simulink library "seriallib"  (Simulink 5.0)
undefined symbols (not defined in the file or in its folder): mbaseserialmask, mmodemcontrol, mquamask, mrs232
libraries: xpclib x193, vxlib x36, simulink x4
(part 2 of 3)

== system seriallib/RS232/Quatech/QSC-200/300 ==
  Modem Control : S-Function  InitFcn=mmodemcontrol(3)  FunctionName=modemcontrolqua  Parameters=slot, port, boardtype, rts, dtr, count  mask(QSC-200/300 Modem Control){port=1, rts=on, dtr=on, slot=-1}
      mask prompts: slot "PCI slot: (-1 for autosearch)"
      mask help:
      | QSC-200/300
      | Quatech
      | Modem Control
      mask init:
      | count = 0;
      | boardtype = 3;
      | [maskdisplay, count] = mmodemcontrol( 2, rts, dtr, boardtype, 0, 0 );
      | set_param( gcb, 'MaskDisplay', maskdisplay );
      mask Help: helpview(fullfile(docroot, 'mapfiles', 'xpc.map'), 'Quatech_MODEM_Control')
      mask StyleString: popup(1|2|3|4),checkbox,checkbox,edit
      mask Display: disp('QSC-200/300\nQuatech\nModem Control');port_label('input',1,'RTS');port_label('input',2,'DTR');
  Modem Status : S-Function  FunctionName=modemstatusqua  Parameters=slot, port, boardtype, cts, dsr, ring, dcd, count, sampletime  mask(Modem Status){port=1, cts=on, dsr=on, ring=on, dcd=on, sampletime=-1, slot=-1}
      mask prompts: ring "RI:"; slot "PCI slot: (-1 for autosearch)"
      mask help:
      | QSC-200/300
      | Quatech
      | Modem Status
      mask init:
      | count = 0;
      | boardtype = 3;
      | [maskdisplay, count] = mmodemstatus( 2, cts, dsr, ring, dcd, boardtype );
      | set_param( gcb, 'MaskDisplay', maskdisplay );
      mask Help: helpview(fullfile(docroot, 'mapfiles', 'xpc.map'), 'Quatech_MODEM_Status')
      mask StyleString: popup(1|2|3|4),checkbox,checkbox,checkbox,checkbox,edit,edit
      mask Display: disp('QSC-200/300\nQuatech\nModem Status');port_label('output',1,'CTS');port_label('output',2,'DSR');port_label('output',3,'RI');port_label('output',4,'DCD');
  QSC-200/300 Internal  blocks1 : Subsystem
  "QSC-200/300 " : Subsystem  InitFcn=mquamask(3)  TreatAsAtomicUnit=on  mask(RS422/485 Send Receive){group=Board Setup, port=1, irqnum=7, slot=-1, baud1=115200, parity1=None, ndata1=8, nstop1=1, fifomode1=64 deep, rlevel1=half full, onxmt1=None, xmtfifosize1=1024, xmtdatatype1=8 bit uint null terminated, rcvfifosize1=1024, rcvmaxread1=1024, rcvminread1=1, rcvusedelim1=on, rcvdelim1=13, rcvdatatype1=count+16 bit uint, rcvsampletime1=-1, baud2=115200, parity2=None, ndata2=8, nstop2=1, fifomode2=64 deep, rlevel2=half full, onxmt2=None, xmtfifosize2=1024, xmtdatatype2=8 bit uint null terminated, rcvfifosize2=1024, rcvmaxread2=1024, rcvminread2=1, rcvusedelim2=on, rcvdelim2=13, rcvdatatype2=count+16 bit uint, rcvsampletime2=-1, baud3=115200, parity3=None, ndata3=8, nstop3=1, fifomode3=64 deep, rlevel3=half full, onxmt3=None, xmtfifosize3=1024, xmtdatatype3=8 bit uint null terminated, rcvfifosize3=1024, rcvmaxread3=1024, rcvminread3=1, rcvusedelim3=on, rcvdelim3=13, rcvdatatype3=count+16 bit uint, rcvsampletime3=-1, buad4=115200, parity4=None, ndata4=8, nstop4=1, fifomode4=64 deep, rlevel4=half full, onxmt4=None, xmtfifosize4=1024, xmtdatatype4=8 bit uint null terminated, rcvfifosize4=1024, rcvmaxread4=1024, rcvminread4=1, rcvusedelim4=on, rcvdelim4=13, rcvdatatype4=count+16 bit uint, rcvsampletime4=-1}
      mask prompts: group "Parameter group:"; port "Port to modify:"; irqnum "IRQ number:"; baud1 "Baud rate:"; parity1 "Parity:"; ndata1 "Data bits:"; nstop1 "Stop bits:"; fifomode1 "Hardware fifo size:"; rlevel1 "Receive fifo interrupt level:"; onxmt1 "Assert on transmit:"; xmtfifosize1 "Transmit software fifo size:"; xmtdatatype1 "Transmit fifo data type:"; rcvfifosize1 "Receive software fifo size:"; rcvmaxread1 "Receive maximum read:"; rcvminread1 "Receive minimum read:"; rcvusedelim1 "Read to delimiter:"; rcvdelim1 "Delimiter:"; rcvdatatype1 "Receive data type:"; rcvsampletime1 "Receive SampleTime:"; baud2 "Baud rate:"; parity2 "Parity:"; ndata2 "Data bits:"; nstop2 "Stop bits:"; fifomode2 "Hardware fifo size:"; rlevel2 "Receive fifo interrupt level:"; onxmt2 "Assert on transmit:"; xmtfifosize2 "Transmit software fifo size:"; xmtdatatype2 "Transmit fifo data type:"; rcvfifosize2 "Receive software fifo size:"; rcvmaxread2 "Receive maximum read:"; rcvminread2 "Receive minimum read:"; rcvusedelim2 "Read to delimiter:"; rcvdelim2 "Delimiter:"; rcvdatatype2 "Receive data type:"; rcvsampletime2 "Receive SampleTime:"; baud3 "Baud rate:"; parity3 "Parity:"; ndata3 "Data bits:"; nstop3 "Stop bits:"; fifomode3 "Hardware fifo size:"; rlevel3 "Receive fifo interrupt level:"; onxmt3 "Assert on transmit:"; xmtfifosize3 "Transmit software fifo size:"; xmtdatatype3 "Transmit fifo data type:"; rcvfifosize3 "Receive software fifo size:"; rcvmaxread3 "Receive maximum read:"; rcvminread3 "Receive minimum read:"; rcvusedelim3 "Read to delimiter:"; rcvdelim3 "Delimiter:"; rcvdatatype3 "Receive data type:"; rcvsampletime3 "Receive SampleTime:"; buad4 "Baud rate:"; parity4 "Parity:"; ndata4 "Data bits:"; nstop4 "Stop bits:"; fifomode4 "Hardware fifo size:"; rlevel4 "Receive fifo interrupt level:"; onxmt4 "Assert on transmit:"; xmtfifosize4 "Transmit software fifo size:"; xmtdatatype4 "Transmit fifo data type:"; rcvfifosize4 "Receive software fifo size:"; rcvmaxread4 "Receive maximum read:"; rcvminread4 "Receive minimum read:"; rcvusedelim4 "Read to delimiter:"; rcvdelim4 "Delimiter:"; rcvdatatype4 "Receive data type:"; rcvsampletime4 "Receive SampleTime:"
      mask help:
      | QSC-200/300
      | Quatech
      | RS422/485 Send Receive Subsystem
      mask init:
      | brdslot = slot;
      | mqua2mask( 1, 4 );
      mask Help: helpview(fullfile(docroot, 'mapfiles', 'xpc.map'), 'Quatech_Subsystem')
      mask StyleString: popup(Board Setup|Basic Setup|Transmit Setup|Receive Setup),popup(1|2|3|4),edit,edit,popup(921600|460800|230400|115200|57600|38400|19200|9600|4800|2400|1200|600|300|110),popup(None|Even|Odd|Mark|Space),popup(5|6|7|8),popup(1|2),popup(64 deep|16 deep|1 deep),popup(1|quarter full|half full|almost full),popup(None|RTS|DTR),edit,popup(count+32 bit int|count+32 bit uint|count+16 bit int|count+16 bit uint|8 bit int null terminated|8 bit uint null terminated),edit,edit,edit,checkbox,edit,popup(count+32 bit int|count+32 bit uint|count+16 bit int|count+16 bit uint|8 bit int null terminated|8 bit uint null terminated),edit,popup(921600|460800|230400|115200|57600|38400|19200|9600|4800|2400|1200|600|300|110),popup(None|Even|Odd|Mark|Space),popup(5|6|7|8),popup(1|2),popup(64 deep|16 deep|1 deep),popup(1|quarter full|half full|almost full),popup(None|RTS|DTR),edit,popup(count+32 bit int|count+32 bit uint|count+16 bit int|count+16 bit uint|8 bit int null terminated|8 bit uint null terminated),edit,edit,edit,checkbox,edit,popup(count+32 bit int|count+32 bit uint|count+16 bit int|count+16 bit uint|8 bit int null terminated|8 bit uint null terminated),edit,popup(921600|460800|230400|115200|57600|38400|19200|9600|4800|2400|1200|600|300|110),popup(None|Even|Odd|Mark|Space),popup(5|6|7|8),popup(1|2),popup(64 deep|16 deep|1 deep),popup(1|quarter full|half full|almost full),popup(None|RTS|DTR),edit,popup(count+32 bit int|count+32 bit uint|count+16 bit int|count+16 bit uint|8 bit int null terminated|8 bit uint null terminated),edit,edit,edit,checkbox,edit,popup(count+32 bit int|count+32 bit uint|count+16 bit int|count+16 bit uint|8 bit int null terminated|8 bit uint null terminated),edit,popup(921600|460800|230400|115200|57600|38400|19200|9600|4800|2400|1200|600|300|110),popup(None|Even|Odd|Mark|Space),popup(5|6|7|8),popup(1|2),popup(64 deep|16 deep|1 deep),popup(1|quarter full|half full|almost full),popup(None|RTS|DTR),edit,popup(count+32 bit int|count+32 bit uint|count+16 bit int|count+16 bit uint|8 bit int null terminated|8 bit uint null terminated),edit,edit,edit,checkbox,edit,popup(count+32 bit int|count+32 bit uint|count+16 bit int|count+16 bit uint|8 bit int null terminated|8 bit uint null terminated),edit
      mask CallbackString:
      | mquamask( 2, 4 );
      | |mquamask( 2, 4 );||||||||||||||||||||||||||||||||||||||||||||||||||||||||||||||||||
      mask Display:
      | disp('QSC-200/300\n\nRS422/485\n\nSend Receive');
      | port_label( 'input', 1, 'XMT1' );
      | port_label( 'input', 2, 'XMT2' );
      | port_label( 'input', 3, 'XMT3' );
      | port_label( 'input', 4, 'XMT4' );
      | port_label( 'output', 1, 'RCV1' );
      | port_label( 'output', 2, 'RCV2' );
      | port_label( 'output', 3, 'RCV3' );
      | port_label( 'output', 4, 'RCV4' );

== system seriallib/RS232/Synchronous Mode/Send & Receive  ==
  In1 : Inport
  S-Function : S-Function  FunctionName=rs232_sendrec  Parameters=port,formatsend,formatrec,numb,ts
  Out1 : Outport
  wires:
  S-Function/1 -> Out1/1
  In1/1 -> S-Function/1

== system seriallib/RS232/Mainboard/Baseboard Serial/RS232 ISR ==
  Xmt 1 : Inport
  Xmt 2 : Inport  Port=2
  function : TriggerPort  TriggerType=function-call
  While Iterator Subsystem : Subsystem  TreatAsAtomicUnit=on
  Recv 1 : Outport
  Recv 2 : Outport  Port=2
  wires:
  While Iterator Subsystem/2(Recv 2) -> Recv 2/1
  While Iterator Subsystem/1(Recv 1) -> Recv 1/1
  Xmt 2/1 -> While Iterator Subsystem/2(Xmt 2)
  Xmt 1/1 -> While Iterator Subsystem/1(Xmt 1)

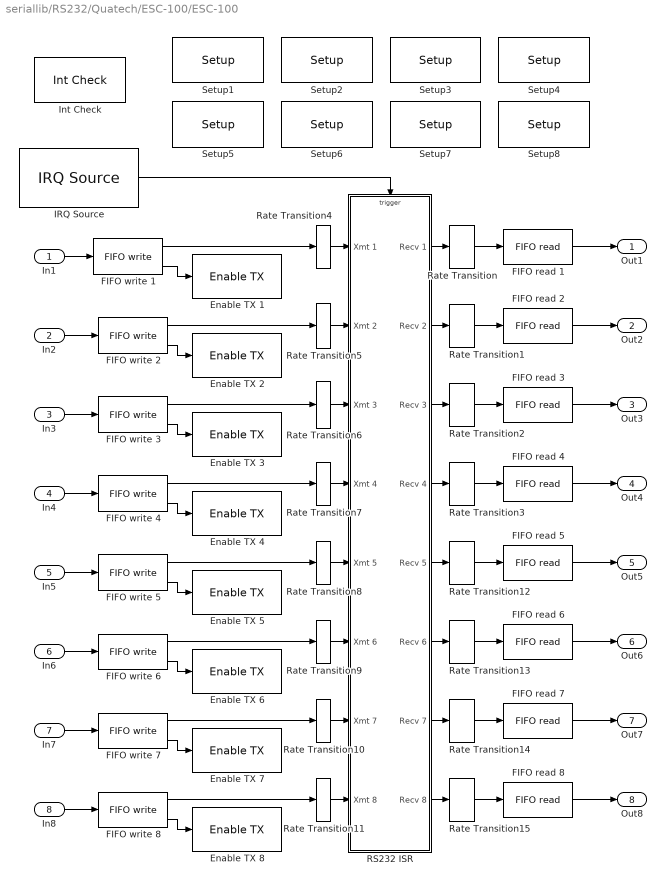
== system seriallib/RS232/Quatech/ESC-100/ESC-100 ==
  In1 : Inport
  In2 : Inport  Port=2
  In3 : Inport  Port=3
  In4 : Inport  Port=4
  In5 : Inport  Port=5
  In6 : Inport  Port=6
  In7 : Inport  Port=7
  In8 : Inport  Port=8
  Enable TX 1 : xpclib/RS232/Quatech/ESC-100/ESC-100 Internal blocks/Enable TX   port=1  slot=brdslot
  Enable TX 2 : xpclib/RS232/Quatech/ESC-100/ESC-100 Internal blocks/Enable TX   port=2  slot=brdslot
  Enable TX 3 : xpclib/RS232/Quatech/ESC-100/ESC-100 Internal blocks/Enable TX   port=3  slot=brdslot
  Enable TX 4 : xpclib/RS232/Quatech/ESC-100/ESC-100 Internal blocks/Enable TX   port=4  slot=brdslot
  Enable TX 5 : xpclib/RS232/Quatech/ESC-100/ESC-100 Internal blocks/Enable TX   port=5  slot=brdslot
  Enable TX 6 : xpclib/RS232/Quatech/ESC-100/ESC-100 Internal blocks/Enable TX   port=6  slot=brdslot
  Enable TX 7 : xpclib/RS232/Quatech/ESC-100/ESC-100 Internal blocks/Enable TX   port=7  slot=brdslot
  Enable TX 8 : xpclib/RS232/Quatech/ESC-100/ESC-100 Internal blocks/Enable TX   port=8  slot=brdslot
  FIFO read {1..8} (8 alike) : xpclib/RS232/FIFO read   maxsize=1024  minsize=1  usedelimiter=on  delimiter=13  outputtype=count+16 bit uint  enable=off  enableout=off  sampletime=-1
  FIFO write {1..8} (8 alike) : xpclib/RS232/FIFO write   size=1024  inputtype=8 bit uint null terminated  present=on  sampletime=-1
  IRQ Source : xpclib/Asynchronous Event/IRQ Source  irqNo=7  preempt=off  b_type=None/Other  slot=brdslot
  Int Check : xpclib/RS232/Quatech/ESC-100/ESC-100 Internal blocks/Int Check  slot=brdslot  irqnum=7
  RS232 ISR : Subsystem  TreatAsAtomicUnit=on  mask(RS232 ISR){slot=brdslot}
      mask help:
      | ESC-100
      | Quatech
      | Interrupt Service Routine
      mask init:
      | subslot = slot;
      mask Display:
      | disp('ESC-100\nISR');
      | port_label('input', 1, 'XMT1');
      | port_label('input', 2, 'XMT2');
      | port_label('input', 3, 'XMT3');
      | port_label('input', 4, 'XMT4');
      | port_label('input', 5, 'XMT5');
      | port_label('input', 6, 'XMT6');
      | port_label('input', 7, 'XMT7');
      | port_label('input', 8, 'XMT8');
      | port_label('output', 1, 'RCV1');
      | port_label('output', 2, 'RCV2');
      | port_label('output', 3, 'RCV3');
      | port_label('output', 4, 'RCV4');
      | port_label('output', 5, 'RCV5');
      | port_label('output', 6, 'RCV6');
      | port_label('output', 7, 'RCV7');
      | port_label('output', 8, 'RCV8');
  Rate Transition{,1..15} (16 alike) : vxlib/Asynchronous Support/Rate Transition  sample_time=-1
  Setup1 : xpclib/RS232/Quatech/ESC-100/ESC-100 Internal blocks/Setup  port=1  baud=19200  width=8  nstop=1  parity=None  fmode=64 deep  rlevel=half full  ctsmode=on  slot=brdslot
  Setup2 : xpclib/RS232/Quatech/ESC-100/ESC-100 Internal blocks/Setup  port=2  baud=19200  width=8  nstop=1  parity=None  fmode=64 deep  rlevel=half full  ctsmode=on  slot=brdslot
  Setup3 : xpclib/RS232/Quatech/ESC-100/ESC-100 Internal blocks/Setup  port=3  baud=19200  width=8  nstop=1  parity=None  fmode=64 deep  rlevel=half full  ctsmode=on  slot=brdslot
  Setup4 : xpclib/RS232/Quatech/ESC-100/ESC-100 Internal blocks/Setup  port=4  baud=19200  width=8  nstop=1  parity=None  fmode=64 deep  rlevel=half full  ctsmode=on  slot=brdslot
  Setup5 : xpclib/RS232/Quatech/ESC-100/ESC-100 Internal blocks/Setup  port=5  baud=19200  width=8  nstop=1  parity=None  fmode=64 deep  rlevel=half full  ctsmode=on  slot=brdslot
  Setup6 : xpclib/RS232/Quatech/ESC-100/ESC-100 Internal blocks/Setup  port=6  baud=19200  width=8  nstop=1  parity=None  fmode=64 deep  rlevel=half full  ctsmode=on  slot=brdslot
  Setup7 : xpclib/RS232/Quatech/ESC-100/ESC-100 Internal blocks/Setup  port=7  baud=19200  width=8  nstop=1  parity=None  fmode=64 deep  rlevel=half full  ctsmode=on  slot=brdslot
  Setup8 : xpclib/RS232/Quatech/ESC-100/ESC-100 Internal blocks/Setup  port=8  baud=19200  width=8  nstop=1  parity=None  fmode=64 deep  rlevel=half full  ctsmode=on  slot=brdslot
  Out1 : Outport
  Out2 : Outport  Port=2
  Out3 : Outport  Port=3
  Out4 : Outport  Port=4
  Out5 : Outport  Port=5
  Out6 : Outport  Port=6
  Out7 : Outport  Port=7
  Out8 : Outport  Port=8
  wires:
  In8/1 -> FIFO write 8/1
  In7/1 -> FIFO write 7/1
  In6/1 -> FIFO write 6/1
  In5/1 -> FIFO write 5/1
  In4/1 -> FIFO write 4/1
  In3/1 -> FIFO write 3/1
  In2/1 -> FIFO write 2/1
  FIFO write 8/2 -> Enable TX 8/1
  FIFO write 7/2 -> Enable TX 7/1
  FIFO write 6/2 -> Enable TX 6/1
  FIFO write 5/2 -> Enable TX 5/1
  FIFO write 4/2 -> Enable TX 4/1
  FIFO write 3/2 -> Enable TX 3/1
  FIFO write 2/2 -> Enable TX 2/1
  FIFO write 8/1 -> Rate Transition11/1
  FIFO write 7/1 -> Rate Transition10/1
  FIFO write 6/1 -> Rate Transition9/1
  FIFO write 5/1 -> Rate Transition8/1
  FIFO write 4/1 -> Rate Transition7/1
  FIFO write 3/1 -> Rate Transition6/1
  FIFO write 2/1 -> Rate Transition5/1
  FIFO write 1/2 -> Enable TX 1/1
  FIFO write 1/1 -> Rate Transition4/1
  In1/1 -> FIFO write 1/1
  IRQ Source/1 -> RS232 ISR/Trigger
  Rate Transition4/1 -> RS232 ISR/1(Xmt 1)
  Rate Transition6/1 -> RS232 ISR/3(Xmt 3)
  Rate Transition7/1 -> RS232 ISR/4(Xmt 4)
  RS232 ISR/1(Recv 1) -> Rate Transition/1
  RS232 ISR/2(Recv 2) -> Rate Transition1/1
  RS232 ISR/3(Recv 3) -> Rate Transition2/1
  Rate Transition/1 -> FIFO read 1/1
  FIFO read 1/1 -> Out1/1
  Rate Transition1/1 -> FIFO read 2/1
  FIFO read 2/1 -> Out2/1
  FIFO read 3/1 -> Out3/1
  FIFO read 4/1 -> Out4/1
  Rate Transition2/1 -> FIFO read 3/1
  Rate Transition3/1 -> FIFO read 4/1
  Rate Transition5/1 -> RS232 ISR/2(Xmt 2)
  RS232 ISR/4(Recv 4) -> Rate Transition3/1
  Rate Transition11/1 -> RS232 ISR/8(Xmt 8)
  Rate Transition10/1 -> RS232 ISR/7(Xmt 7)
  Rate Transition9/1 -> RS232 ISR/6(Xmt 6)
  Rate Transition8/1 -> RS232 ISR/5(Xmt 5)
  FIFO read 5/1 -> Out5/1
  Rate Transition12/1 -> FIFO read 5/1
  FIFO read 6/1 -> Out6/1
  Rate Transition13/1 -> FIFO read 6/1
  FIFO read 7/1 -> Out7/1
  Rate Transition14/1 -> FIFO read 7/1
  FIFO read 8/1 -> Out8/1
  Rate Transition15/1 -> FIFO read 8/1
  RS232 ISR/5(Recv 5) -> Rate Transition12/1
  RS232 ISR/6(Recv 6) -> Rate Transition13/1
  RS232 ISR/7(Recv 7) -> Rate Transition14/1
  RS232 ISR/8(Recv 8) -> Rate Transition15/1

== system seriallib/RS232/Quatech/ESC-100/ESC-100 Internal blocks ==
  "Enable TX " : S-Function  FunctionName=sertxenable  Parameters=slot, port, 2  mask(Enable TX Int){port=1, slot=-1}
      mask prompts: slot "PCI slot: (-1 for autosearch)"
      mask help:
      | ESC-100
      | Quatech
      | Enable TX Interrupt
      mask Help: helpview(fullfile(docroot, 'mapfiles', 'xpc.map'), 'Quatech_Enable_Int')
      mask StyleString: popup(1|2|3|4|5|6|7|8),edit
      mask Display:
      | disp('ESC-100\nQuatech\nEnable TX int');
      | port_label('input', 1, 'E');
  Filter Int Reason : S-Function  FunctionName=filterqua  Parameters=port, 2, value  mask(Interrupt Source Filter){port=1, value=Transmitter empty}
      mask prompts: value "Filter value:"
      mask help:
      | ESC-100
      | Quatech
      | Interrupt Source Filter
      mask Help: helpview(fullfile(docroot, 'mapfiles', 'xpc.map'), 'Quatech_Filter_Ints')
      mask StyleString: popup(1|2|3|4|5|6|7|8),popup(Receive data|Transmitter empty|Modem status change)
      mask Display:
      | disp('ESC-100\nQuatech\nFilter Int Reason');
      | port_label('input', 1, 'S' );
      | port_label('output', 1, 'E' );
  Int Check : S-Function  FunctionName=intcheckqua  Parameters=slot, irqnum+4, boardtype,  mask(interrupt check){slot=-1, irqnum=5}
      mask prompts: slot "PCI slot: (-1 for autosearch)"; irqnum "IRQ Line Number"
      mask help:
      | ESC-100
      | Quatech
      | Interrupt Check
      mask init:
      | boardtype = 2;
      mask Help: helpview(fullfile(docroot, 'mapfiles', 'xpc.map'), 'Quatech_Interrupt_Check')
      mask StyleString: edit,popup(5|6|7|8|9|10|11|12|13|14|15)
      mask Display: disp('ESC-100\nQuatech\nInterrupt Check');
  Read HW FIFO : S-Function  FunctionName=serreadqua  Parameters=slot, port, 2, flush  mask(Read Data Port){port=1, flush=on, slot=-1}
      mask prompts: flush "Flush HW FIFO on startup"; slot "PCI slot: (-1 for autosearch)"
      mask help:
      | ESC-100
      | Quatech
      | Read Data Port
      mask Help: helpview(fullfile(docroot, 'mapfiles', 'xpc.map'), 'Quatech_Read_HW')
      mask StyleString: popup(1|2|3|4|5|6|7|8),checkbox,edit
      mask Display:
      | disp('ESC-100\nQuatech\nRead HW FIFO');
      | port_label('input', 1, 'E');
      | port_label('output', 1, 'D');
  Read Int Status : S-Function  FunctionName=Iqueryqua  Parameters=slot, 2  mask(Interrupt Query){slot=-1}
      mask prompts: slot "PCI slot: (-1 for autosearch)"
      mask help:
      | ESC-100
      | Quatech
      | Interrupt Query
      mask Help: helpview(fullfile(docroot, 'mapfiles', 'xpc.map'), 'Quatech_Interrupt_Query')
      mask Display:
      | disp('ESC-100\nQuatech\nRead Int Status');
      | port_label('output', 1, 'S' );
  Setup : S-Function  FunctionName=setupqua  Parameters=slot, boardtype, port, baud, width, nstop, parity, fmode, ctsmode, rlevel  mask(setup){port=1, baud=115200, width=8, nstop=1, parity=None, fmode=64 deep, rlevel=half full, ctsmode=off, slot=-1}
      mask prompts: baud "Baud rate:"; width "Number of data bits:"; nstop "Number of stop bits:"; fmode "Fifo mode:"; rlevel "Receive trigger level:"; ctsmode "Enable auto RTS/CTS"; slot "PCI slot: (-1 for autosearch)"
      mask help:
      | ESC-100
      | Quatech
      | Setup
      mask init:
      | boardtype = 2;
      mask Help: helpview(fullfile(docroot, 'mapfiles', 'xpc.map'), 'Quatech_Setup')
      mask StyleString: popup(1|2|3|4|5|6|7|8),popup(921600|460800|230400|115200|57600|38400|19200|9600|4800|2400|1200|600|300|110),popup(5|6|7|8),popup(1|2),popup(None|Even|Odd|Mark|Space),popup(64 deep|16 deep|1 deep),popup(1|quarter full|half full|almost full),checkbox,edit
      mask Display: disp('ESC-100\nQuatech\nSetup')
  Write HW FIFO : S-Function  FunctionName=serwritequa  Parameters=slot, port, 2, 0  mask(Write Data Port){port=1, slot=-1}
      mask prompts: slot "PCI slot: (-1 for autosearch)"
      mask help:
      | ESC-100
      | Quatech
      | Write Data Port
      mask Help: helpview(fullfile(docroot, 'mapfiles', 'xpc.map'), 'Quatech_Write_HW')
      mask StyleString: popup(1|2|3|4|5|6|7|8),edit
      mask Display:
      | disp('ESC-100\nQuatech\nWrite HW FIFO');
      | port_label('input', 1, 'D');
      | port_label('input', 2, 'E');

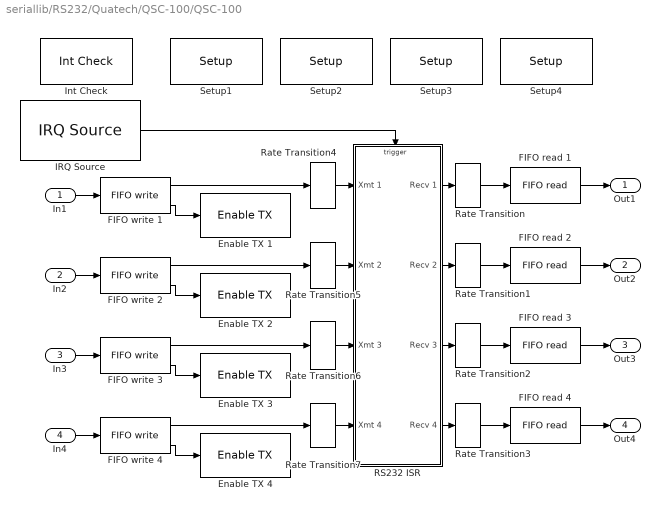
== system seriallib/RS232/Quatech/QSC-100/QSC-100 ==
  In1 : Inport
  In2 : Inport  Port=2
  In3 : Inport  Port=3
  In4 : Inport  Port=4
  Enable TX 1 : xpclib/RS232/Quatech/QSC-100/QSC-100 Internal  blocks/Enable TX   port=1  slot=brdslot
  Enable TX 2 : xpclib/RS232/Quatech/QSC-100/QSC-100 Internal  blocks/Enable TX   port=2  slot=brdslot
  Enable TX 3 : xpclib/RS232/Quatech/QSC-100/QSC-100 Internal  blocks/Enable TX   port=3  slot=brdslot
  Enable TX 4 : xpclib/RS232/Quatech/QSC-100/QSC-100 Internal  blocks/Enable TX   port=4  slot=brdslot
  FIFO read {1..4} (4 alike) : xpclib/RS232/FIFO read   maxsize=1024  minsize=1  usedelimiter=on  delimiter=13  outputtype=count+16 bit uint  enable=off  enableout=off  sampletime=-1
  FIFO write {1..4} (4 alike) : xpclib/RS232/FIFO write   size=1024  inputtype=8 bit uint null terminated  present=on  sampletime=-1
  IRQ Source : xpclib/Asynchronous Event/IRQ Source  irqNo=7  preempt=off  b_type=None/Other  slot=brdslot
  Int Check : xpclib/RS232/Quatech/QSC-100/QSC-100 Internal  blocks/Int Check  slot=brdslot  irqnum=7
  RS232 ISR : Subsystem  TreatAsAtomicUnit=on  mask(RS232 ISR){slot=brdslot}
      mask help:
      | QSC-100
      | Quatech
      | Interrupt Service Routine
      mask init:
      | subslot = slot;
      mask Display:
      | disp('QSC-100\nISR');
      | port_label('input', 1, 'XMT1');
      | port_label('input', 2, 'XMT2');
      | port_label('input', 3, 'XMT3');
      | port_label('input', 4, 'XMT4');
      | port_label('output', 1, 'RCV1');
      | port_label('output', 2, 'RCV2');
      | port_label('output', 3, 'RCV3');
      | port_label('output', 4, 'RCV4');
  Rate Transition{,1..7} (8 alike) : vxlib/Asynchronous Support/Rate Transition  sample_time=-1
  Setup1 : xpclib/RS232/Quatech/QSC-100/QSC-100 Internal  blocks/Setup  port=1  baud=115200  width=8  nstop=1  parity=None  fmode=64 deep  rlevel=half full  ctsmode=on  slot=brdslot
  Setup2 : xpclib/RS232/Quatech/QSC-100/QSC-100 Internal  blocks/Setup  port=2  baud=115200  width=8  nstop=1  parity=None  fmode=64 deep  rlevel=half full  ctsmode=on  slot=brdslot
  Setup3 : xpclib/RS232/Quatech/QSC-100/QSC-100 Internal  blocks/Setup  port=3  baud=115200  width=8  nstop=1  parity=None  fmode=64 deep  rlevel=half full  ctsmode=on  slot=brdslot
  Setup4 : xpclib/RS232/Quatech/QSC-100/QSC-100 Internal  blocks/Setup  port=4  baud=115200  width=8  nstop=1  parity=None  fmode=64 deep  rlevel=half full  ctsmode=on  slot=brdslot
  Out1 : Outport
  Out2 : Outport  Port=2
  Out3 : Outport  Port=3
  Out4 : Outport  Port=4
  wires:
  RS232 ISR/4(Recv 4) -> Rate Transition3/1
  Rate Transition5/1 -> RS232 ISR/2(Xmt 2)
  FIFO write 4/2 -> Enable TX 4/1
  FIFO write 3/2 -> Enable TX 3/1
  FIFO write 2/2 -> Enable TX 2/1
  Rate Transition3/1 -> FIFO read 4/1
  Rate Transition2/1 -> FIFO read 3/1
  FIFO read 4/1 -> Out4/1
  FIFO read 3/1 -> Out3/1
  FIFO read 2/1 -> Out2/1
  Rate Transition1/1 -> FIFO read 2/1
  FIFO read 1/1 -> Out1/1
  Rate Transition/1 -> FIFO read 1/1
  In2/1 -> FIFO write 2/1
  In3/1 -> FIFO write 3/1
  In4/1 -> FIFO write 4/1
  FIFO write 4/1 -> Rate Transition7/1
  FIFO write 3/1 -> Rate Transition6/1
  FIFO write 2/1 -> Rate Transition5/1
  In1/1 -> FIFO write 1/1
  FIFO write 1/1 -> Rate Transition4/1
  RS232 ISR/3(Recv 3) -> Rate Transition2/1
  RS232 ISR/2(Recv 2) -> Rate Transition1/1
  RS232 ISR/1(Recv 1) -> Rate Transition/1
  Rate Transition7/1 -> RS232 ISR/4(Xmt 4)
  Rate Transition6/1 -> RS232 ISR/3(Xmt 3)
  Rate Transition4/1 -> RS232 ISR/1(Xmt 1)
  IRQ Source/1 -> RS232 ISR/Trigger
  FIFO write 1/2 -> Enable TX 1/1

== system seriallib/RS232/Quatech/QSC-100/QSC-100 Internal  blocks ==
  "Enable TX " : S-Function  FunctionName=sertxenable  Parameters=slot, port, 1  mask(Enable TX Int){port=1, slot=-1}
      mask prompts: slot "PCI slot: (-1 for autosearch)"
      mask help:
      | QSC-100
      | Quatech
      | Enable TX Interrupt
      mask Help: helpview(fullfile(docroot, 'mapfiles', 'xpc.map'), 'Quatech_Enable_Int')
      mask StyleString: popup(1|2|3|4),edit
      mask Display:
      | disp('QSC-100\nQuatech\nEnable TX int');
      | port_label('input', 1, 'E');
  Filter Int Reason : S-Function  FunctionName=filterqua  Parameters=port, 1, value  mask(Interrupt Source Filter){port=1, value=Receive data}
      mask prompts: value "Filter value:"
      mask help:
      | QSC-100
      | Quatech
      | Interrupt Source Filter
      mask Help: helpview(fullfile(docroot, 'mapfiles', 'xpc.map'), 'Quatech_Filter_Ints')
      mask StyleString: popup(1|2|3|4),popup(Receive data|Transmitter empty|Modem status change)
      mask Display:
      | disp('QSC-100\nQuatech\nFilter Int Reason');
      | port_label('input', 1, 'S' );
      | port_label('output', 1, 'E' );
  Int Check : S-Function  FunctionName=intcheckqua  Parameters=slot, irqnum+4, boardtype,  mask(interrupt check){slot=-1, irqnum=5}
      mask prompts: slot "PCI slot: (-1 for autosearch)"; irqnum "IRQ Line Number"
      mask help:
      | QSC-100
      | Quatech
      | Interrupt Check
      mask init:
      | boardtype = 1;
      mask Help: helpview(fullfile(docroot, 'mapfiles', 'xpc.map'), 'Quatech_Interrupt_Check')
      mask StyleString: edit,popup(5|6|7|8|9|10|11|12|13|14|15)
      mask Display: disp('QSC-100\nQuatech\nInterrupt Check');
  Read HW FIFO : S-Function  FunctionName=serreadqua  Parameters=slot, port, 1, flush  mask(Read Data Port){port=1, flush=on, slot=-1}
      mask prompts: flush "Flush HW FIFO on startup"; slot "PCI slot: (-1 for autosearch)"
      mask help:
      | QSC-100
      | Quatech
      | Read Data Port
      mask Help: helpview(fullfile(docroot, 'mapfiles', 'xpc.map'), 'Quatech_Read_HW')
      mask StyleString: popup(1|2|3|4),checkbox,edit
      mask Display:
      | disp('QSC-100\nQuatech\nRead HW FIFO');
      | port_label('input', 1, 'E');
      | port_label('output', 1, 'D');
  Read Int Status : S-Function  FunctionName=Iqueryqua  Parameters=slot, 1  mask(Interrupt Query){slot=-1}
      mask prompts: slot "PCI slot: (-1 for autosearch)"
      mask help:
      | QSC-100
      | Quatech
      | Interrupt Query
      mask Help: helpview(fullfile(docroot, 'mapfiles', 'xpc.map'), 'Quatech_Interrupt_Query')
      mask Display:
      | disp('QSC-100\nQuatech\nRead Int Status');
      | port_label('output', 1, 'S' );
  Setup : S-Function  FunctionName=setupqua  Parameters=slot, boardtype, port, baud, width, nstop, parity, fmode, ctsmode, rlevel  mask(setup){port=1, baud=115200, width=8, nstop=1, parity=None, fmode=64 deep, rlevel=half full, ctsmode=off, slot=-1}
      mask prompts: baud "Baud rate:"; width "Number of data bits:"; nstop "Number of stop bits:"; fmode "Fifo mode:"; rlevel "Receive trigger level:"; ctsmode "Enable auto RTS/CTS"; slot "PCI slot: (-1 for autosearch)"
      mask help:
      | QSC-100
      | Quatech
      | Setup
      mask init:
      | boardtype = 1;
      mask Help: helpview(fullfile(docroot, 'mapfiles', 'xpc.map'), 'Quatech_Setup')
      mask StyleString: popup(1|2|3|4),popup(921600|460800|230400|115200|57600|38400|19200|9600|4800|2400|1200|600|300|110),popup(5|6|7|8),popup(1|2),popup(None|Even|Odd|Mark|Space),popup(64 deep|16 deep|1 deep),popup(1|quarter full|half full|almost full),checkbox,edit
      mask Display: disp('QSC-100\nQuatech\nSetup');
  Write HW FIFO : S-Function  FunctionName=serwritequa  Parameters=slot, port, 1, 0  mask(Write Data Port){port=1, slot=-1}
      mask prompts: slot "PCI slot: (-1 for autosearch)"
      mask help:
      | QSC-100
      | Quatech
      | Write Data Port
      mask Help: helpview(fullfile(docroot, 'mapfiles', 'xpc.map'), 'Quatech_Write_HW')
      mask StyleString: popup(1|2|3|4),edit
      mask Display:
      | disp('QSC-100\nQuatech\nWrite HW FIFO');
      | port_label('input', 1, 'D');
      | port_label('input', 2, 'E');

== system seriallib/RS232/Quatech/QSC-200/300/QSC-200/300 Internal  blocks1 ==
  "Enable TX " : S-Function  FunctionName=sertxenable  Parameters=slot, port, 3  mask(Enable TX Int){port=1, slot=-1}
      mask prompts: slot "PCI slot: (-1 for autosearch)"
      mask help:
      | QSC-200/300
      | Quatech
      | Enable TX Interrupt
      mask Help: helpview(fullfile(docroot, 'mapfiles', 'xpc.map'), 'Quatech_Enable_Int')
      mask StyleString: popup(1|2|3|4),edit
      mask Display:
      | disp('QSC-200/300\nQuatech\nEnable TX int');
      | port_label('input', 1, 'E');
  Filter Int Reason : S-Function  FunctionName=filterqua  Parameters=port, 3, value  mask(Interrupt Source Filter){port=1, value=Receive data}
      mask prompts: value "Filter value:"
      mask help:
      | QSC-200/300
      | Quatech
      | Interrupt Source Filter
      mask Help: helpview(fullfile(docroot, 'mapfiles', 'xpc.map'), 'Quatech_Filter_Ints')
      mask StyleString: popup(1|2|3|4),popup(Receive data|Transmitter empty|Modem status change)
      mask Display:
      | disp('QSC-200/300\nQuatech\nFilter Int Reason');
      | port_label('input', 1, 'S' );
      | port_label('output', 1, 'E' );
  Int Check : S-Function  FunctionName=intcheckqua  Parameters=slot, irqnum+4, boardtype,  mask(interrupt check){slot=-1, irqnum=5}
      mask prompts: slot "PCI slot: (-1 for autosearch)"; irqnum "IRQ Line Number"
      mask help:
      | QSC-200/300
      | Quatech
      | Interrupt Check
      mask init:
      | boardtype = 3;
      mask Help: helpview(fullfile(docroot, 'mapfiles', 'xpc.map'), 'Quatech_Interrupt_Check')
      mask StyleString: edit,popup(5|6|7|8|9|10|11|12|13|14|15)
      mask Display: disp('QSC-200/300\nQuatech\nInterrupt Check');
  Read HW FIFO : S-Function  FunctionName=serreadqua  Parameters=slot, port, 3, flush  mask(Read Data Port){port=1, flush=on, slot=-1}
      mask prompts: flush "Flush HW FIFO on startup"; slot "PCI slot: (-1 for autosearch)"
      mask help:
      | QSC-200/300
      | Quatech
      | Read Data Port
      mask Help: helpview(fullfile(docroot, 'mapfiles', 'xpc.map'), 'Quatech_Read_HW')
      mask StyleString: popup(1|2|3|4),checkbox,edit
      mask Display:
      | disp('QSC-200/300\nQuatech\nRead HW FIFO');
      | port_label('input', 1, 'E');
      | port_label('output', 1, 'D');
  Read Int Status : S-Function  FunctionName=Iqueryqua  Parameters=slot, 3  mask(Interrupt Query){slot=-1}
      mask prompts: slot "PCI slot: (-1 for autosearch)"
      mask help:
      | QSC-200/300
      | Quatech
      | Interrupt Query
      mask Help: helpview(fullfile(docroot, 'mapfiles', 'xpc.map'), 'Quatech_Interrupt_Query')
      mask Display:
      | disp('QSC-200/300\nQuatech\nRead Int Status');
      | port_label('output', 1, 'S' );
  Setup : S-Function  FunctionName=setupqua  Parameters=slot, boardtype, port, baud, width, nstop, parity, fmode, ctsmode, rlevel  mask(setup){port=1, baud=115200, width=8, nstop=1, parity=None, fmode=64 deep, rlevel=half full, ctsmode=off, slot=-1}
      mask prompts: baud "Baud rate:"; width "Number of data bits:"; nstop "Number of stop bits:"; fmode "Fifo mode:"; rlevel "Receive trigger level:"; ctsmode "Enable auto RTS/CTS"; slot "PCI slot: (-1 for autosearch)"
      mask help:
      | QSC-200/300
      | Quatech
      | Setup
      mask init:
      | boardtype = 3;
      mask Help: helpview(fullfile(docroot, 'mapfiles', 'xpc.map'), 'Quatech_Setup')
      mask StyleString: popup(1|2|3|4),popup(921600|460800|230400|115200|57600|38400|19200|9600|4800|2400|1200|600|300|110),popup(5|6|7|8),popup(1|2),popup(None|Even|Odd|Mark|Space),popup(64 deep|16 deep|1 deep),popup(1|quarter full|half full|almost full),checkbox,edit
      mask Display: disp('QSC-200/300\nQuatech\nSetup');
  Write HW FIFO : S-Function  FunctionName=serwritequa  Parameters=slot, port, 3, onxmt  mask(Write Data Port){port=1, onxmt=None, slot=-1}
      mask prompts: onxmt "Assert on Transmit:"; slot "PCI slot: (-1 for autosearch)"
      mask help:
      | QSC-200/300
      | Quatech
      | Write Data Port
      mask Help: helpview(fullfile(docroot, 'mapfiles', 'xpc.map'), 'Quatech_Write_HW')
      mask StyleString: popup(1|2|3|4),popup(None|RTS|DTR),edit
      mask Display:
      | disp('QSC-200/300\nQuatech\nWrite HW FIFO');
      | port_label('input', 1, 'D');
      | port_label('input', 2, 'E');

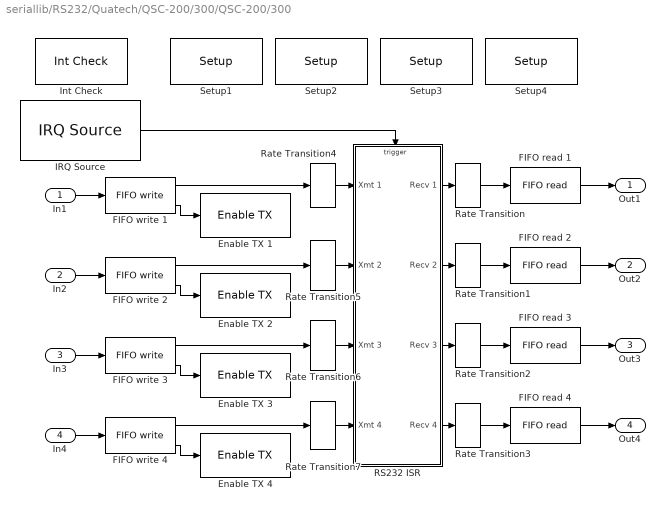
== system seriallib/RS232/Quatech/QSC-200/300/QSC-200/300  ==
  In1 : Inport
  In2 : Inport  Port=2
  In3 : Inport  Port=3
  In4 : Inport  Port=4
  Enable TX 1 : xpclib/RS232/Quatech/QSC-200//300/QSC-200//300 Internal  blocks1/Enable TX   port=1  slot=brdslot
  Enable TX 2 : xpclib/RS232/Quatech/QSC-200//300/QSC-200//300 Internal  blocks1/Enable TX   port=2  slot=brdslot
  Enable TX 3 : xpclib/RS232/Quatech/QSC-200//300/QSC-200//300 Internal  blocks1/Enable TX   port=3  slot=brdslot
  Enable TX 4 : xpclib/RS232/Quatech/QSC-200//300/QSC-200//300 Internal  blocks1/Enable TX   port=4  slot=brdslot
  FIFO read {1..4} (4 alike) : xpclib/RS232/FIFO read   maxsize=1024  minsize=1  usedelimiter=on  delimiter=13  outputtype=count+16 bit uint  enable=off  enableout=off  sampletime=-1
  FIFO write {1..4} (4 alike) : xpclib/RS232/FIFO write   size=1024  inputtype=8 bit uint null terminated  present=on  sampletime=-1
  IRQ Source : xpclib/Asynchronous Event/IRQ Source  irqNo=7  preempt=off  b_type=None/Other  slot=brdslot
  Int Check : xpclib/RS232/Quatech/QSC-200//300/QSC-200//300 Internal  blocks1/Int Check  slot=brdslot  irqnum=7
  RS232 ISR : Subsystem  TreatAsAtomicUnit=on  mask(RS232 ISR){slot=brdslot}
      mask help:
      | QSC-100
      | Quatech
      | Interrupt Service Routine
      mask init:
      | subslot = slot;
      mask Display:
      | disp('QSC-100\nISR');
      | port_label('input', 1, 'XMT1');
      | port_label('input', 2, 'XMT2');
      | port_label('input', 3, 'XMT3');
      | port_label('input', 4, 'XMT4');
      | port_label('output', 1, 'RCV1');
      | port_label('output', 2, 'RCV2');
      | port_label('output', 3, 'RCV3');
      | port_label('output', 4, 'RCV4');
  Rate Transition{,1..7} (8 alike) : vxlib/Asynchronous Support/Rate Transition  sample_time=-1
  Setup1 : xpclib/RS232/Quatech/QSC-200//300/QSC-200//300 Internal  blocks1/Setup  port=1  baud=115200  width=8  nstop=1  parity=None  fmode=64 deep  rlevel=half full  ctsmode=on  slot=brdslot
  Setup2 : xpclib/RS232/Quatech/QSC-200//300/QSC-200//300 Internal  blocks1/Setup  port=2  baud=115200  width=8  nstop=1  parity=None  fmode=64 deep  rlevel=half full  ctsmode=on  slot=brdslot
  Setup3 : xpclib/RS232/Quatech/QSC-200//300/QSC-200//300 Internal  blocks1/Setup  port=3  baud=115200  width=8  nstop=1  parity=None  fmode=64 deep  rlevel=half full  ctsmode=on  slot=brdslot
  Setup4 : xpclib/RS232/Quatech/QSC-200//300/QSC-200//300 Internal  blocks1/Setup  port=4  baud=115200  width=8  nstop=1  parity=None  fmode=64 deep  rlevel=half full  ctsmode=on  slot=brdslot
  Out1 : Outport
  Out2 : Outport  Port=2
  Out3 : Outport  Port=3
  Out4 : Outport  Port=4
  wires:
  FIFO write 1/2 -> Enable TX 1/1
  IRQ Source/1 -> RS232 ISR/Trigger
  Rate Transition4/1 -> RS232 ISR/1(Xmt 1)
  Rate Transition6/1 -> RS232 ISR/3(Xmt 3)
  Rate Transition7/1 -> RS232 ISR/4(Xmt 4)
  RS232 ISR/1(Recv 1) -> Rate Transition/1
  RS232 ISR/2(Recv 2) -> Rate Transition1/1
  RS232 ISR/3(Recv 3) -> Rate Transition2/1
  FIFO write 1/1 -> Rate Transition4/1
  In1/1 -> FIFO write 1/1
  FIFO write 2/1 -> Rate Transition5/1
  FIFO write 3/1 -> Rate Transition6/1
  FIFO write 4/1 -> Rate Transition7/1
  In4/1 -> FIFO write 4/1
  In3/1 -> FIFO write 3/1
  In2/1 -> FIFO write 2/1
  Rate Transition/1 -> FIFO read 1/1
  FIFO read 1/1 -> Out1/1
  Rate Transition1/1 -> FIFO read 2/1
  FIFO read 2/1 -> Out2/1
  FIFO read 3/1 -> Out3/1
  FIFO read 4/1 -> Out4/1
  Rate Transition2/1 -> FIFO read 3/1
  Rate Transition3/1 -> FIFO read 4/1
  FIFO write 2/2 -> Enable TX 2/1
  FIFO write 3/2 -> Enable TX 3/1
  FIFO write 4/2 -> Enable TX 4/1
  Rate Transition5/1 -> RS232 ISR/2(Xmt 2)
  RS232 ISR/4(Recv 4) -> Rate Transition3/1

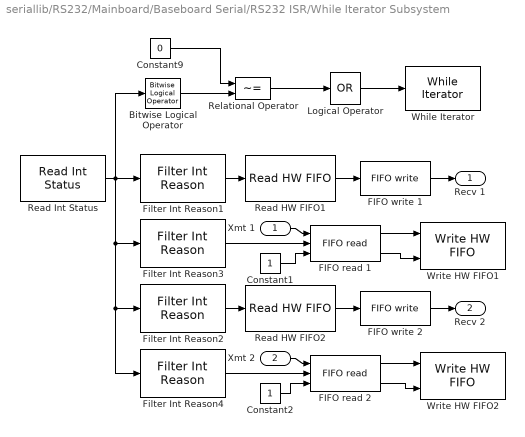
== system seriallib/RS232/Mainboard/Baseboard Serial/RS232 ISR/While Iterator Subsystem ==
  Xmt 1 : Inport
  Xmt 2 : Inport  Port=2
  Bitwise Logical Operator : simulink/Math Operations/Bitwise Logical Operator  Operator=AND  Operand2='FF'
  Constant1 : Constant  ShowAdditionalParam=on  OutDataTypeMode=uint32
  Constant2 : Constant  ShowAdditionalParam=on  OutDataTypeMode=uint32
  Constant9 : Constant  Value=0  ShowAdditionalParam=on  OutDataTypeMode=uint32
  FIFO read 1 : xpclib/RS232/FIFO read   maxsize=60  minsize=1  usedelimiter=off  delimiter=13  outputtype=count+32 bit uint  enable=on  enableout=on  sampletime=-1
  FIFO read 2 : xpclib/RS232/FIFO read   maxsize=60  minsize=1  usedelimiter=off  delimiter=13  outputtype=count+32 bit uint  enable=on  enableout=on  sampletime=-1
  FIFO write 1 : xpclib/RS232/FIFO write   size=1024  inputtype=count+32 bit uint  present=off  sampletime=-1
  FIFO write 2 : xpclib/RS232/FIFO write   size=1024  inputtype=count+32 bit uint  present=off  sampletime=-1
  Filter Int Reason1 : xpclib/RS232/Mainboard/Baseboard Serial Internal  blocks/Filter Int Reason  port=1  value=Receive data
  Filter Int Reason2 : xpclib/RS232/Mainboard/Baseboard Serial Internal  blocks/Filter Int Reason  port=2  value=Receive data
  Filter Int Reason3 : xpclib/RS232/Mainboard/Baseboard Serial Internal  blocks/Filter Int Reason  port=1  value=Transmitter empty
  Filter Int Reason4 : xpclib/RS232/Mainboard/Baseboard Serial Internal  blocks/Filter Int Reason  port=2  value=Transmitter empty
  Logical Operator : Logic  Operator=OR  Inputs=1  AllPortsSameDT=off
  Read HW FIFO1 : xpclib/RS232/Mainboard/Baseboard Serial Internal  blocks/Read HW FIFO  flush=on  addr=baddr1
  Read HW FIFO2 : xpclib/RS232/Mainboard/Baseboard Serial Internal  blocks/Read HW FIFO  flush=on  addr=baddr2
  Read Int Status : xpclib/RS232/Mainboard/Baseboard Serial Internal  blocks/Read Int Status  addr1=baddr1  addr2=baddr2
  Relational Operator : RelationalOperator  Operator=~=
  While Iterator : WhileIterator  MaxIters=65  WhileBlockType=do-while
  Write HW FIFO1 : xpclib/RS232/Mainboard/Baseboard Serial Internal  blocks/Write HW FIFO  addr=baddr1
  Write HW FIFO2 : xpclib/RS232/Mainboard/Baseboard Serial Internal  blocks/Write HW FIFO  addr=baddr2
  Recv 1 : Outport
  Recv 2 : Outport  Port=2
  wires:
  Constant9/1 -> Relational Operator/1
  Bitwise Logical Operator/1 -> Relational Operator/2
  Relational Operator/1 -> Logical Operator/1
  Logical Operator/1 -> While Iterator/1
  Constant2/1 -> FIFO read 2/3
  Constant1/1 -> FIFO read 1/3
  FIFO read 1/2 -> Write HW FIFO1/2
  FIFO read 1/1 -> Write HW FIFO1/1
  FIFO read 2/2 -> Write HW FIFO2/2
  FIFO read 2/1 -> Write HW FIFO2/1
  Xmt 2/1 -> FIFO read 2/1
  Filter Int Reason4/1 -> FIFO read 2/2
  Read HW FIFO2/1 -> FIFO write 2/1
  FIFO write 2/1 -> Recv 2/1
  Filter Int Reason2/1 -> Read HW FIFO2/1
  Xmt 1/1 -> FIFO read 1/1
  Filter Int Reason3/1 -> FIFO read 1/2
  Read HW FIFO1/1 -> FIFO write 1/1
  FIFO write 1/1 -> Recv 1/1
  Filter Int Reason1/1 -> Read HW FIFO1/1
  Read Int Status/1 -> Bitwise Logical Operator/1, Filter Int Reason2/1, Filter Int Reason4/1, Filter Int Reason3/1, Filter Int Reason1/1

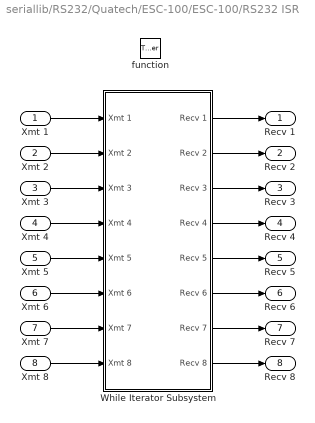
== system seriallib/RS232/Quatech/ESC-100/ESC-100/RS232 ISR ==
  Xmt 1 : Inport
  Xmt 2 : Inport  Port=2
  Xmt 3 : Inport  Port=3
  Xmt 4 : Inport  Port=4
  Xmt 5 : Inport  Port=5
  Xmt 6 : Inport  Port=6
  Xmt 7 : Inport  Port=7
  Xmt 8 : Inport  Port=8
  function : TriggerPort  TriggerType=function-call
  While Iterator Subsystem : Subsystem  TreatAsAtomicUnit=on
  Recv 1 : Outport
  Recv 2 : Outport  Port=2
  Recv 3 : Outport  Port=3
  Recv 4 : Outport  Port=4
  Recv 5 : Outport  Port=5
  Recv 6 : Outport  Port=6
  Recv 7 : Outport  Port=7
  Recv 8 : Outport  Port=8
  wires:
  While Iterator Subsystem/8(Recv 8) -> Recv 8/1
  While Iterator Subsystem/7(Recv 7) -> Recv 7/1
  While Iterator Subsystem/6(Recv 6) -> Recv 6/1
  While Iterator Subsystem/5(Recv 5) -> Recv 5/1
  While Iterator Subsystem/4(Recv 4) -> Recv 4/1
  While Iterator Subsystem/3(Recv 3) -> Recv 3/1
  While Iterator Subsystem/2(Recv 2) -> Recv 2/1
  While Iterator Subsystem/1(Recv 1) -> Recv 1/1
  Xmt 8/1 -> While Iterator Subsystem/8(Xmt 8)
  Xmt 7/1 -> While Iterator Subsystem/7(Xmt 7)
  Xmt 6/1 -> While Iterator Subsystem/6(Xmt 6)
  Xmt 5/1 -> While Iterator Subsystem/5(Xmt 5)
  Xmt 4/1 -> While Iterator Subsystem/4(Xmt 4)
  Xmt 3/1 -> While Iterator Subsystem/3(Xmt 3)
  Xmt 2/1 -> While Iterator Subsystem/2(Xmt 2)
  Xmt 1/1 -> While Iterator Subsystem/1(Xmt 1)

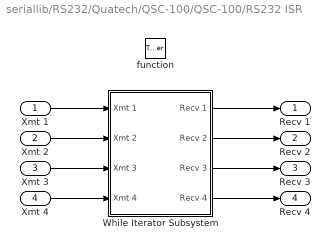
== system seriallib/RS232/Quatech/QSC-100/QSC-100/RS232 ISR ==
  Xmt 1 : Inport
  Xmt 2 : Inport  Port=2
  Xmt 3 : Inport  Port=3
  Xmt 4 : Inport  Port=4
  function : TriggerPort  TriggerType=function-call
  While Iterator Subsystem : Subsystem  TreatAsAtomicUnit=on
  Recv 1 : Outport
  Recv 2 : Outport  Port=2
  Recv 3 : Outport  Port=3
  Recv 4 : Outport  Port=4
  wires:
  While Iterator Subsystem/4(Recv 4) -> Recv 4/1
  While Iterator Subsystem/3(Recv 3) -> Recv 3/1
  While Iterator Subsystem/2(Recv 2) -> Recv 2/1
  While Iterator Subsystem/1(Recv 1) -> Recv 1/1
  Xmt 4/1 -> While Iterator Subsystem/4(Xmt 4)
  Xmt 3/1 -> While Iterator Subsystem/3(Xmt 3)
  Xmt 2/1 -> While Iterator Subsystem/2(Xmt 2)
  Xmt 1/1 -> While Iterator Subsystem/1(Xmt 1)

== system seriallib/RS232/Quatech/QSC-200/300/QSC-200/300 /RS232 ISR ==
  Xmt 1 : Inport
  Xmt 2 : Inport  Port=2
  Xmt 3 : Inport  Port=3
  Xmt 4 : Inport  Port=4
  function : TriggerPort  TriggerType=function-call
  While Iterator Subsystem : Subsystem  TreatAsAtomicUnit=on
  Recv 1 : Outport
  Recv 2 : Outport  Port=2
  Recv 3 : Outport  Port=3
  Recv 4 : Outport  Port=4
  wires:
  While Iterator Subsystem/4(Recv 4) -> Recv 4/1
  While Iterator Subsystem/3(Recv 3) -> Recv 3/1
  While Iterator Subsystem/2(Recv 2) -> Recv 2/1
  While Iterator Subsystem/1(Recv 1) -> Recv 1/1
  Xmt 4/1 -> While Iterator Subsystem/4(Xmt 4)
  Xmt 3/1 -> While Iterator Subsystem/3(Xmt 3)
  Xmt 2/1 -> While Iterator Subsystem/2(Xmt 2)
  Xmt 1/1 -> While Iterator Subsystem/1(Xmt 1)

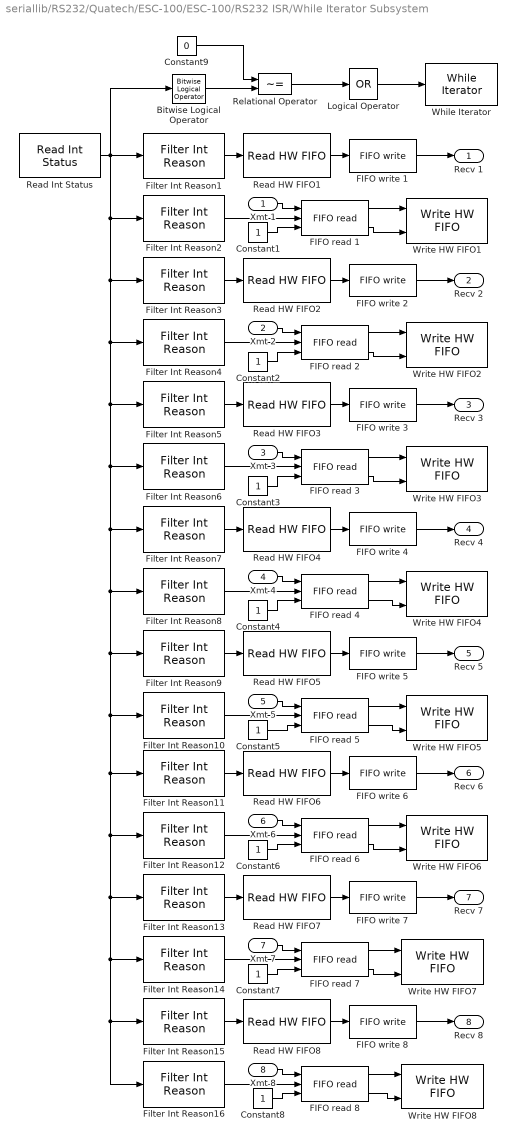
== system seriallib/RS232/Quatech/ESC-100/ESC-100/RS232 ISR/While Iterator Subsystem ==
  Xmt 1 : Inport
  Xmt 2 : Inport  Port=2
  Xmt 3 : Inport  Port=3
  Xmt 4 : Inport  Port=4
  Xmt 5 : Inport  Port=5
  Xmt 6 : Inport  Port=6
  Xmt 7 : Inport  Port=7
  Xmt 8 : Inport  Port=8
  Bitwise Logical Operator : simulink/Math Operations/Bitwise Logical Operator  Operator=AND  Operand2='FF'
  Constant{1..8} (8 alike) : Constant  ShowAdditionalParam=on  OutDataTypeMode=uint32
  Constant9 : Constant  Value=0  ShowAdditionalParam=on  OutDataTypeMode=uint32
  FIFO read {1..8} (8 alike) : xpclib/RS232/FIFO read   maxsize=60  minsize=1  usedelimiter=off  delimiter=13  outputtype=count+32 bit uint  enable=on  enableout=on  sampletime=-1
  FIFO write {1..8} (8 alike) : xpclib/RS232/FIFO write   size=1024  inputtype=count+32 bit uint  present=off  sampletime=-1
  Filter Int Reason1 : xpclib/RS232/Quatech/ESC-100/ESC-100 Internal blocks/Filter Int Reason  port=1  value=Receive data
  Filter Int Reason10 : xpclib/RS232/Quatech/ESC-100/ESC-100 Internal blocks/Filter Int Reason  port=5  value=Transmitter empty
  Filter Int Reason11 : xpclib/RS232/Quatech/ESC-100/ESC-100 Internal blocks/Filter Int Reason  port=6  value=Receive data
  Filter Int Reason12 : xpclib/RS232/Quatech/ESC-100/ESC-100 Internal blocks/Filter Int Reason  port=6  value=Transmitter empty
  Filter Int Reason13 : xpclib/RS232/Quatech/ESC-100/ESC-100 Internal blocks/Filter Int Reason  port=7  value=Receive data
  Filter Int Reason14 : xpclib/RS232/Quatech/ESC-100/ESC-100 Internal blocks/Filter Int Reason  port=7  value=Transmitter empty
  Filter Int Reason15 : xpclib/RS232/Quatech/ESC-100/ESC-100 Internal blocks/Filter Int Reason  port=8  value=Receive data
  Filter Int Reason16 : xpclib/RS232/Quatech/ESC-100/ESC-100 Internal blocks/Filter Int Reason  port=8  value=Transmitter empty
  Filter Int Reason2 : xpclib/RS232/Quatech/ESC-100/ESC-100 Internal blocks/Filter Int Reason  port=1  value=Transmitter empty
  Filter Int Reason3 : xpclib/RS232/Quatech/ESC-100/ESC-100 Internal blocks/Filter Int Reason  port=2  value=Receive data
  Filter Int Reason4 : xpclib/RS232/Quatech/ESC-100/ESC-100 Internal blocks/Filter Int Reason  port=2  value=Transmitter empty
  Filter Int Reason5 : xpclib/RS232/Quatech/ESC-100/ESC-100 Internal blocks/Filter Int Reason  port=3  value=Receive data
  Filter Int Reason6 : xpclib/RS232/Quatech/ESC-100/ESC-100 Internal blocks/Filter Int Reason  port=3  value=Transmitter empty
  Filter Int Reason7 : xpclib/RS232/Quatech/ESC-100/ESC-100 Internal blocks/Filter Int Reason  port=4  value=Receive data
  Filter Int Reason8 : xpclib/RS232/Quatech/ESC-100/ESC-100 Internal blocks/Filter Int Reason  port=4  value=Transmitter empty
  Filter Int Reason9 : xpclib/RS232/Quatech/ESC-100/ESC-100 Internal blocks/Filter Int Reason  port=5  value=Receive data
  Logical Operator : Logic  Operator=OR  Inputs=1  AllPortsSameDT=off
  Read HW FIFO1 : xpclib/RS232/Quatech/ESC-100/ESC-100 Internal blocks/Read HW FIFO  port=1  flush=on  slot=subslot
  Read HW FIFO2 : xpclib/RS232/Quatech/ESC-100/ESC-100 Internal blocks/Read HW FIFO  port=2  flush=on  slot=subslot
  Read HW FIFO3 : xpclib/RS232/Quatech/ESC-100/ESC-100 Internal blocks/Read HW FIFO  port=3  flush=on  slot=subslot
  Read HW FIFO4 : xpclib/RS232/Quatech/ESC-100/ESC-100 Internal blocks/Read HW FIFO  port=4  flush=on  slot=subslot
  Read HW FIFO5 : xpclib/RS232/Quatech/ESC-100/ESC-100 Internal blocks/Read HW FIFO  port=5  flush=on  slot=subslot
  Read HW FIFO6 : xpclib/RS232/Quatech/ESC-100/ESC-100 Internal blocks/Read HW FIFO  port=6  flush=on  slot=subslot
  Read HW FIFO7 : xpclib/RS232/Quatech/ESC-100/ESC-100 Internal blocks/Read HW FIFO  port=7  flush=on  slot=subslot
  Read HW FIFO8 : xpclib/RS232/Quatech/ESC-100/ESC-100 Internal blocks/Read HW FIFO  port=8  flush=on  slot=subslot
  Read Int Status : xpclib/RS232/Quatech/ESC-100/ESC-100 Internal blocks/Read Int Status  slot=subslot
  Relational Operator : RelationalOperator  Operator=~=
  While Iterator : WhileIterator  MaxIters=65  WhileBlockType=do-while
  Write HW FIFO1 : xpclib/RS232/Quatech/ESC-100/ESC-100 Internal blocks/Write HW FIFO  port=1  slot=subslot
  Write HW FIFO2 : xpclib/RS232/Quatech/ESC-100/ESC-100 Internal blocks/Write HW FIFO  port=2  slot=subslot
  Write HW FIFO3 : xpclib/RS232/Quatech/ESC-100/ESC-100 Internal blocks/Write HW FIFO  port=3  slot=subslot
  Write HW FIFO4 : xpclib/RS232/Quatech/ESC-100/ESC-100 Internal blocks/Write HW FIFO  port=4  slot=subslot
  Write HW FIFO5 : xpclib/RS232/Quatech/ESC-100/ESC-100 Internal blocks/Write HW FIFO  port=5  slot=subslot
  Write HW FIFO6 : xpclib/RS232/Quatech/ESC-100/ESC-100 Internal blocks/Write HW FIFO  port=6  slot=subslot
  Write HW FIFO7 : xpclib/RS232/Quatech/ESC-100/ESC-100 Internal blocks/Write HW FIFO  port=7  slot=subslot
  Write HW FIFO8 : xpclib/RS232/Quatech/ESC-100/ESC-100 Internal blocks/Write HW FIFO  port=8  slot=subslot
  Recv 1 : Outport
  Recv 2 : Outport  Port=2
  Recv 3 : Outport  Port=3
  Recv 4 : Outport  Port=4
  Recv 5 : Outport  Port=5
  Recv 6 : Outport  Port=6
  Recv 7 : Outport  Port=7
  Recv 8 : Outport  Port=8
  wires:
  Constant9/1 -> Relational Operator/1
  Bitwise Logical Operator/1 -> Relational Operator/2
  Relational Operator/1 -> Logical Operator/1
  Logical Operator/1 -> While Iterator/1
  Constant8/1 -> FIFO read 8/3
  Constant7/1 -> FIFO read 7/3
  Constant6/1 -> FIFO read 6/3
  Constant5/1 -> FIFO read 5/3
  Constant4/1 -> FIFO read 4/3
  Constant3/1 -> FIFO read 3/3
  Constant2/1 -> FIFO read 2/3
  Constant1/1 -> FIFO read 1/3
  FIFO read 1/2 -> Write HW FIFO1/2
  FIFO read 1/1 -> Write HW FIFO1/1
  FIFO read 2/2 -> Write HW FIFO2/2
  FIFO read 2/1 -> Write HW FIFO2/1
  FIFO read 3/2 -> Write HW FIFO3/2
  FIFO read 3/1 -> Write HW FIFO3/1
  FIFO read 4/2 -> Write HW FIFO4/2
  FIFO read 4/1 -> Write HW FIFO4/1
  FIFO read 5/2 -> Write HW FIFO5/2
  FIFO read 5/1 -> Write HW FIFO5/1
  FIFO read 6/2 -> Write HW FIFO6/2
  FIFO read 6/1 -> Write HW FIFO6/1
  FIFO read 7/2 -> Write HW FIFO7/2
  FIFO read 7/1 -> Write HW FIFO7/1
  FIFO read 8/2 -> Write HW FIFO8/2
  FIFO read 8/1 -> Write HW FIFO8/1
  Xmt 8/1 -> FIFO read 8/1
  Filter Int Reason16/1 -> FIFO read 8/2
  Read HW FIFO8/1 -> FIFO write 8/1
  FIFO write 8/1 -> Recv 8/1
  Filter Int Reason15/1 -> Read HW FIFO8/1
  Xmt 7/1 -> FIFO read 7/1
  Filter Int Reason14/1 -> FIFO read 7/2
  Read HW FIFO7/1 -> FIFO write 7/1
  FIFO write 7/1 -> Recv 7/1
  Filter Int Reason13/1 -> Read HW FIFO7/1
  Xmt 6/1 -> FIFO read 6/1
  Filter Int Reason12/1 -> FIFO read 6/2
  Read HW FIFO6/1 -> FIFO write 6/1
  FIFO write 6/1 -> Recv 6/1
  Filter Int Reason11/1 -> Read HW FIFO6/1
  Xmt 5/1 -> FIFO read 5/1
  Filter Int Reason10/1 -> FIFO read 5/2
  Read HW FIFO5/1 -> FIFO write 5/1
  FIFO write 5/1 -> Recv 5/1
  Filter Int Reason9/1 -> Read HW FIFO5/1
  Xmt 4/1 -> FIFO read 4/1
  Filter Int Reason8/1 -> FIFO read 4/2
  Read HW FIFO4/1 -> FIFO write 4/1
  FIFO write 4/1 -> Recv 4/1
  Filter Int Reason7/1 -> Read HW FIFO4/1
  Xmt 3/1 -> FIFO read 3/1
  Filter Int Reason6/1 -> FIFO read 3/2
  Read HW FIFO3/1 -> FIFO write 3/1
  FIFO write 3/1 -> Recv 3/1
  Filter Int Reason5/1 -> Read HW FIFO3/1
  Xmt 2/1 -> FIFO read 2/1
  Filter Int Reason4/1 -> FIFO read 2/2
  Read HW FIFO2/1 -> FIFO write 2/1
  FIFO write 2/1 -> Recv 2/1
  Filter Int Reason3/1 -> Read HW FIFO2/1
  Xmt 1/1 -> FIFO read 1/1
  Filter Int Reason2/1 -> FIFO read 1/2
  Read HW FIFO1/1 -> FIFO write 1/1
  FIFO write 1/1 -> Recv 1/1
  Filter Int Reason1/1 -> Read HW FIFO1/1
  Read Int Status/1 -> Bitwise Logical Operator/1, Filter Int Reason15/1, Filter Int Reason16/1, Filter Int Reason14/1, Filter Int Reason13/1, Filter Int Reason12/1, Filter Int Reason11/1, Filter Int Reason10/1, Filter Int Reason9/1, Filter Int Reason8/1, Filter Int Reason7/1, Filter Int Reason6/1, Filter Int Reason5/1, Filter Int Reason4/1, Filter Int Reason3/1, Filter Int Reason2/1, Filter Int Reason1/1
